simulink library "inp_BCKP"  (R2021b)
settings: Solver=VariableStepAuto  StartTime=0.0  StopTime=10.0  RelTol=1e-3
undefined symbols (not defined in the file): C_TASK_5MS_S, FALSE, KINP_AcoreReadyToSlp_flg_ovrdflg, KINP_AcoreReadyToSlp_flg_ovrdval, KINP_AllowMovThd_OTA_enum_ovrdflg, KINP_AllowMovThd_OTA_enum_ovrdval, KINP_APSAngleTarget_Deg_ovrdflg, KINP_APSAngleTarget_Deg_ovrdval, KINP_APSDecReq_mps2_ovrdflg, KINP_APSDecReq_mps2_ovrdval, KINP_APSDecReqA_flg_ovrdflg, KINP_APSDecReqA_flg_ovrdval, KINP_APSDFLL_cm_ovrdflg, KINP_APSDFLL_cm_ovrdval, KINP_APSDFLR_cm_ovrdflg, KINP_APSDFLR_cm_ovrdval, KINP_APSDRLL_cm_ovrdflg, KINP_APSDRLL_cm_ovrdval, KINP_APSDRLR_cm_ovrdflg, KINP_APSDRLR_cm_ovrdval, KINP_APSExitCondition_enum_ovrdflg, KINP_APSExitCondition_enum_ovrdval, KINP_APSHWVer_enum_ovrdflg, KINP_APSHWVer_enum_ovrdval, KINP_APSProgressPCT_pct_ovrdflg, KINP_APSProgressPCT_pct_ovrdval, KINP_APSPwrReq_enum_ovrdflg, KINP_APSPwrReq_enum_ovrdval, KINP_APSReq_enum_ovrdflg, KINP_APSReq_enum_ovrdval, KINP_APSRQDisplay_enum_ovrdflg, KINP_APSRQDisplay_enum_ovrdval, KINP_APSRqEPASCtrl_flg_ovrdflg, KINP_APSRqEPASCtrl_flg_ovrdval, KINP_APSShiftPosnReq_enum_ovrdval, KINP_APSShiftPosnReq_enum_ovrflg, KINP_APSSpeedCMD_kph_ovrdval, KINP_APSSpeedCMD_kph_ovrflg, KINP_APSStaSystem_enum_ovrdflg, KINP_APSStaSystem_enum_ovrdval, KINP_APSSWVer_enum_ovrdflg, KINP_APSSWVer_enum_ovrdval, KINP_APSVMCReqA_flg_ovrdval, KINP_APSVMCReqA_flg_ovrflg, KINP_APSVRqEPASCtrl_flg_ovrdflg, KINP_APSVRqEPASCtrl_flg_ovrdval, KINP_AuxBattVolmV_mV_ovrdflg, KINP_AuxBattVolmV_mV_ovrdval, KINP_BTConnectSta_enum_ovrdflg, KINP_BTConnectSta_enum_ovrdval, KINP_CAASSta_enum_ovrdflg, KINP_CAASSta_enum_ovrdval, KINP_CAASVMCReqA_flg_ovrdval, KINP_CAASVMCReqA_flg_ovrflg, KINP_CAN1BusOff_flg_ovrdflg, KINP_CAN1BusOff_flg_ovrdval, KINP_CAN2BusOff_flg_ovrdflg, KINP_CAN2BusOff_flg_ovrdval, KINP_CAN3BusOff_flg_ovrdflg, KINP_CAN3BusOff_flg_ovrdval ... (+158)
libraries: FVT_lib x144, hcu_lib x1
(part 8 of 8)

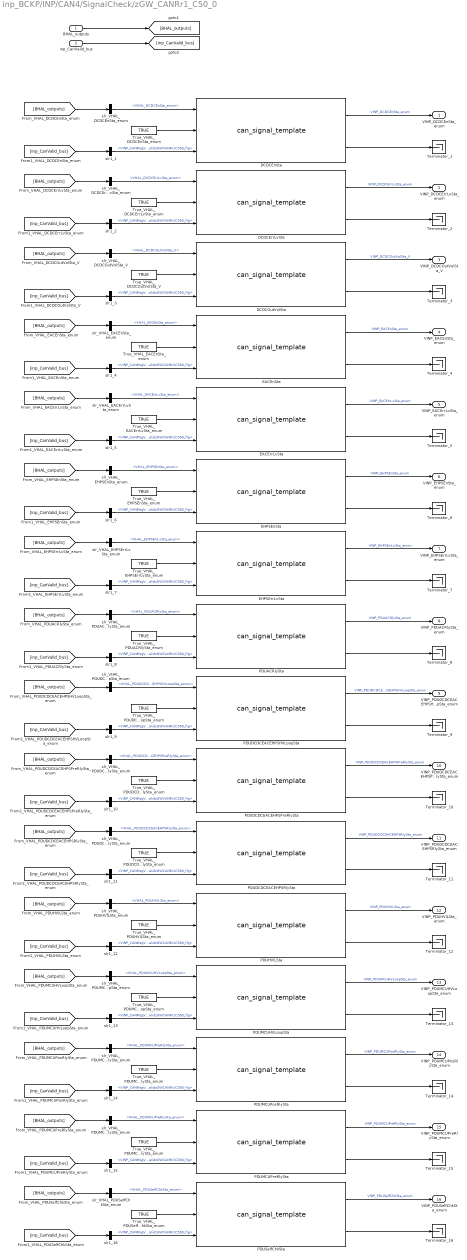
== system inp_BCKP/INP/CAN4/SignalCheck/zGW_CANRr1_C50_0 ==
  BHAL_outputs : Inport
  inp_CanValid_bus : Inport  Port=2
  DCDCEnSta : FVT_lib/inp/can_signal_template  SystemSampleTime=-1  VariantActivationTime=update diagram  Latency=0  AutoFrameSizeCalculation=off
      link override defval: Value=KINP_DCDCEnSta_enum_defval
      link override ovrdflg: Value=KINP_DCDCEnSta_enum_ovrdflg
      link override ovrdval: Value=KINP_DCDCEnSta_enum_ovrdval
  DCDCErrLvSta : FVT_lib/inp/can_signal_template  SystemSampleTime=-1  VariantActivationTime=update diagram  Latency=0  AutoFrameSizeCalculation=off
      link override defval: Value=KINP_DCDCErrLvSta_enum_defval
      link override ovrdflg: Value=KINP_DCDCErrLvSta_enum_ovrdflg
      link override ovrdval: Value=KINP_DCDCErrLvSta_enum_ovrdval
  DCDCOutVolSta : FVT_lib/inp/can_signal_template  SystemSampleTime=-1  VariantActivationTime=update diagram  Latency=0  AutoFrameSizeCalculation=off
      link override defval: Value=KINP_DCDCOutVolSta_V_defval
      link override ovrdflg: Value=KINP_DCDCOutVolSta_V_ovrdflg
      link override ovrdval: Value=KINP_DCDCOutVolSta_V_ovrdval
  EACEnSta : FVT_lib/inp/can_signal_template  SystemSampleTime=-1  VariantActivationTime=update diagram  Latency=0  AutoFrameSizeCalculation=off
      link override defval: Value=KINP_EACEnSta_enum_defval
      link override ovrdflg: Value=KINP_EACEnSta_enum_ovrdflg
      link override ovrdval: Value=KINP_EACEnSta_enum_ovrdval
  EACErrLvSta : FVT_lib/inp/can_signal_template  SystemSampleTime=-1  VariantActivationTime=update diagram  Latency=0  AutoFrameSizeCalculation=off
      link override defval: Value=KINP_EACErrLvSta_enum_defval
      link override ovrdflg: Value=KINP_EACErrLvSta_enum_ovrdflg
      link override ovrdval: Value=KINP_EACErrLvSta_enum_ovrdval
  EHPSEnSta : FVT_lib/inp/can_signal_template  SystemSampleTime=-1  VariantActivationTime=update diagram  Latency=0  AutoFrameSizeCalculation=off
      link override defval: Value=KINP_EHPSEnSta_enum_defval
      link override ovrdflg: Value=KINP_EHPSEnSta_enum_ovrdflg
      link override ovrdval: Value=KINP_EHPSEnSta_enum_ovrdval
  EHPSErrLvSta : FVT_lib/inp/can_signal_template  SystemSampleTime=-1  VariantActivationTime=update diagram  Latency=0  AutoFrameSizeCalculation=off
      link override defval: Value=KINP_EHPSErrLvSta_enum_defval
      link override ovrdflg: Value=KINP_EHPSErrLvSta_enum_ovrdflg
      link override ovrdval: Value=KINP_EHPSErrLvSta_enum_ovrdval
  PDUACRlySta : FVT_lib/inp/can_signal_template  SystemSampleTime=-1  VariantActivationTime=update diagram  Latency=0  AutoFrameSizeCalculation=off
      link override defval: Value=KINP_PDUACRlySta_enum_defval
      link override ovrdflg: Value=KINP_PDUACRlySta_enum_ovrdflg
      link override ovrdval: Value=KINP_PDUACRlySta_enum_ovrdval
  PDUDCDCEACEHPSHVLoopSta : FVT_lib/inp/can_signal_template  SystemSampleTime=-1  VariantActivationTime=update diagram  Latency=0  AutoFrameSizeCalculation=off
      link override defval: Value=KINP_PDUDCDCEACEHPSHVLoopSta_enum_defval
      link override ovrdflg: Value=KINP_PDUDCDCEACEHPSHVLoopSta_enum_ovrdflg
      link override ovrdval: Value=KINP_PDUDCDCEACEHPSHVLoopSta_enum_ovrdval
  PDUDCDCEACEHPSPreRlySta : FVT_lib/inp/can_signal_template  SystemSampleTime=-1  VariantActivationTime=update diagram  Latency=0  AutoFrameSizeCalculation=off
      link override defval: Value=KINP_PDUDCDCEACEHPSPreRlySta_enum_defval
      link override ovrdflg: Value=KINP_PDUDCDCEACEHPSPreRlySta_enum_ovrdflg
      link override ovrdval: Value=KINP_PDUDCDCEACEHPSPreRlySta_enum_ovrdval
  PDUDCDCEACEHPSRlySta : FVT_lib/inp/can_signal_template  SystemSampleTime=-1  VariantActivationTime=update diagram  Latency=0  AutoFrameSizeCalculation=off
      link override defval: Value=KINP_PDUDCDCEACEHPSRlySta_enum_defval
      link override ovrdflg: Value=KINP_PDUDCDCEACEHPSRlySta_enum_ovrdflg
      link override ovrdval: Value=KINP_PDUDCDCEACEHPSRlySta_enum_ovrdval
  PDUHVILSta : FVT_lib/inp/can_signal_template  SystemSampleTime=-1  VariantActivationTime=update diagram  Latency=0  AutoFrameSizeCalculation=off
      link override defval: Value=KINP_PDUHVILSta_enum_defval
      link override ovrdflg: Value=KINP_PDUHVILSta_enum_ovrdflg
      link override ovrdval: Value=KINP_PDUHVILSta_enum_ovrdval
  PDUMCUHVLoopSta : FVT_lib/inp/can_signal_template  SystemSampleTime=-1  VariantActivationTime=update diagram  Latency=0  AutoFrameSizeCalculation=off
      link override defval: Value=KINP_PDUMCUHVLoopSta_enum_defval
      link override ovrdflg: Value=KINP_PDUMCUHVLoopSta_enum_ovrdflg
      link override ovrdval: Value=KINP_PDUMCUHVLoopSta_enum_ovrdval
  PDUMCUPosRlySta : FVT_lib/inp/can_signal_template  SystemSampleTime=-1  VariantActivationTime=update diagram  Latency=0  AutoFrameSizeCalculation=off
      link override defval: Value=KINP_PDUMCUPosRlySta_enum_defval
      link override ovrdflg: Value=KINP_PDUMCUPosRlySta_enum_ovrdflg
      link override ovrdval: Value=KINP_PDUMCUPosRlySta_enum_ovrdval
  PDUMCUPreRlySta : FVT_lib/inp/can_signal_template  SystemSampleTime=-1  VariantActivationTime=update diagram  Latency=0  AutoFrameSizeCalculation=off
      link override defval: Value=KINP_PDUMCUPreRlySta_enum_defval
      link override ovrdflg: Value=KINP_PDUMCUPreRlySta_enum_ovrdflg
      link override ovrdval: Value=KINP_PDUMCUPreRlySta_enum_ovrdval
  PDUSelfChkSta : FVT_lib/inp/can_signal_template  SystemSampleTime=-1  VariantActivationTime=update diagram  Latency=0  AutoFrameSizeCalculation=off
      link override defval: Value=KINP_PDUSelfChkSta_enum_defval
      link override ovrdflg: Value=KINP_PDUSelfChkSta_enum_ovrdflg
      link override ovrdval: Value=KINP_PDUSelfChkSta_enum_ovrdval
  Terminator_{1..16} (16 alike) : Terminator
  True_VHAL_DCDCEnSta_enum : Constant  Value=TRUE  OutDataTypeStr=boolean
  True_VHAL_DCDCErrLvSta_enum : Constant  Value=TRUE  OutDataTypeStr=boolean
  True_VHAL_DCDCOutVolSta_V : Constant  Value=TRUE  OutDataTypeStr=boolean
  True_VHAL_EACEnSta_enum : Constant  Value=TRUE  OutDataTypeStr=boolean
  True_VHAL_EACErrLvSta_enum : Constant  Value=TRUE  OutDataTypeStr=boolean
  True_VHAL_EHPSEnSta_enum : Constant  Value=TRUE  OutDataTypeStr=boolean
  True_VHAL_EHPSErrLvSta_enum : Constant  Value=TRUE  OutDataTypeStr=boolean
  True_VHAL_PDUACRlySta_enum : Constant  Value=TRUE  OutDataTypeStr=boolean
  True_VHAL_PDUDCDCEACEHPSHVLoopSta_enum : Constant  Value=TRUE  OutDataTypeStr=boolean
  True_VHAL_PDUDCDCEACEHPSPreRlySta_enum : Constant  Value=TRUE  OutDataTypeStr=boolean
  True_VHAL_PDUDCDCEACEHPSRlySta_enum : Constant  Value=TRUE  OutDataTypeStr=boolean
  True_VHAL_PDUHVILSta_enum : Constant  Value=TRUE  OutDataTypeStr=boolean
  True_VHAL_PDUMCUHVLoopSta_enum : Constant  Value=TRUE  OutDataTypeStr=boolean
  True_VHAL_PDUMCUPosRlySta_enum : Constant  Value=TRUE  OutDataTypeStr=boolean
  True_VHAL_PDUMCUPreRlySta_enum : Constant  Value=TRUE  OutDataTypeStr=boolean
  True_VHAL_PDUSelfChkSta_enum : Constant  Value=TRUE  OutDataTypeStr=boolean
  slr1_{1..16} (16 alike) : BusSelector  OutputSignals=VINP_CANMsgValidzGWCANRr1C500_flg
  slr_VHAL_DCDCEnSta_enum : BusSelector  OutputSignals=VHAL_DCDCEnSta_enum
  slr_VHAL_DCDCErrLvSta_enum : BusSelector  OutputSignals=VHAL_DCDCErrLvSta_enum
  slr_VHAL_DCDCOutVolSta_V : BusSelector  OutputSignals=VHAL_DCDCOutVolSta_V
  slr_VHAL_EACEnSta_enum : BusSelector  OutputSignals=VHAL_EACEnSta_enum
  slr_VHAL_EACErrLvSta_enum : BusSelector  OutputSignals=VHAL_EACErrLvSta_enum
  slr_VHAL_EHPSEnSta_enum : BusSelector  OutputSignals=VHAL_EHPSEnSta_enum
  slr_VHAL_EHPSErrLvSta_enum : BusSelector  OutputSignals=VHAL_EHPSErrLvSta_enum
  slr_VHAL_PDUACRlySta_enum : BusSelector  OutputSignals=VHAL_PDUACRlySta_enum
  slr_VHAL_PDUDCDCEACEHPSHVLoopSta_enum : BusSelector  OutputSignals=VHAL_PDUDCDCEACEHPSHVLoopSta_enum
  slr_VHAL_PDUDCDCEACEHPSPreRlySta_enum : BusSelector  OutputSignals=VHAL_PDUDCDCEACEHPSPreRlySta_enum
  slr_VHAL_PDUDCDCEACEHPSRlySta_enum : BusSelector  OutputSignals=VHAL_PDUDCDCEACEHPSRlySta_enum
  slr_VHAL_PDUHVILSta_enum : BusSelector  OutputSignals=VHAL_PDUHVILSta_enum
  slr_VHAL_PDUMCUHVLoopSta_enum : BusSelector  OutputSignals=VHAL_PDUMCUHVLoopSta_enum
  slr_VHAL_PDUMCUPosRlySta_enum : BusSelector  OutputSignals=VHAL_PDUMCUPosRlySta_enum
  slr_VHAL_PDUMCUPreRlySta_enum : BusSelector  OutputSignals=VHAL_PDUMCUPreRlySta_enum
  slr_VHAL_PDUSelfChkSta_enum : BusSelector  OutputSignals=VHAL_PDUSelfChkSta_enum
  VINP_DCDCEnSta_enum : Outport
  VINP_DCDCErrLvSta_enum : Outport  Port=2
  VINP_DCDCOutVolSta_V : Outport  Port=3
  VINP_EACEnSta_enum : Outport  Port=4
  VINP_EACErrLvSta_enum : Outport  Port=5
  VINP_EHPSEnSta_enum : Outport  Port=6
  VINP_EHPSErrLvSta_enum : Outport  Port=7
  VINP_PDUACRlySta_enum : Outport  Port=8
  VINP_PDUDCDCEACEHPSHVLoopSta_enum : Outport  Port=9
  VINP_PDUDCDCEACEHPSPreRlySta_enum : Outport  Port=10
  VINP_PDUDCDCEACEHPSRlySta_enum : Outport  Port=11
  VINP_PDUHVILSta_enum : Outport  Port=12
  VINP_PDUMCUHVLoopSta_enum : Outport  Port=13
  VINP_PDUMCUPosRlySta_enum : Outport  Port=14
  VINP_PDUMCUPreRlySta_enum : Outport  Port=15
  VINP_PDUSelfChkSta_enum : Outport  Port=16
  wires:
  BHAL_outputs/1 -> [BHAL_outputs]
  inp_CanValid_bus/1 -> [inp_CanValid_bus]
  [BHAL_outputs] -> slr_VHAL_DCDCEnSta_enum/1
  slr_VHAL_DCDCEnSta_enum/1 -> DCDCEnSta/1  "<VHAL_DCDCEnSta_enum>"
  True_VHAL_DCDCEnSta_enum/1 -> DCDCEnSta/2
  [inp_CanValid_bus] -> slr1_1/1
  slr1_1/1 -> DCDCEnSta/3  "<VINP_CANMsgValidzGWCANRr1C500_flg>"
  DCDCEnSta/1 -> VINP_DCDCEnSta_enum/1  "VINP_DCDCEnSta_enum"
  DCDCEnSta/2 -> Terminator_1/1
  [BHAL_outputs] -> slr_VHAL_DCDCErrLvSta_enum/1
  slr_VHAL_DCDCErrLvSta_enum/1 -> DCDCErrLvSta/1  "<VHAL_DCDCErrLvSta_enum>"
  True_VHAL_DCDCErrLvSta_enum/1 -> DCDCErrLvSta/2
  [inp_CanValid_bus] -> slr1_2/1
  slr1_2/1 -> DCDCErrLvSta/3  "<VINP_CANMsgValidzGWCANRr1C500_flg>"
  DCDCErrLvSta/1 -> VINP_DCDCErrLvSta_enum/1  "VINP_DCDCErrLvSta_enum"
  DCDCErrLvSta/2 -> Terminator_2/1
  [BHAL_outputs] -> slr_VHAL_DCDCOutVolSta_V/1
  slr_VHAL_DCDCOutVolSta_V/1 -> DCDCOutVolSta/1  "<VHAL_DCDCOutVolSta_V>"
  True_VHAL_DCDCOutVolSta_V/1 -> DCDCOutVolSta/2
  [inp_CanValid_bus] -> slr1_3/1
  slr1_3/1 -> DCDCOutVolSta/3  "<VINP_CANMsgValidzGWCANRr1C500_flg>"
  DCDCOutVolSta/1 -> VINP_DCDCOutVolSta_V/1  "VINP_DCDCOutVolSta_V"
  DCDCOutVolSta/2 -> Terminator_3/1
  [BHAL_outputs] -> slr_VHAL_EACEnSta_enum/1
  slr_VHAL_EACEnSta_enum/1 -> EACEnSta/1  "<VHAL_EACEnSta_enum>"
  True_VHAL_EACEnSta_enum/1 -> EACEnSta/2
  [inp_CanValid_bus] -> slr1_4/1
  slr1_4/1 -> EACEnSta/3  "<VINP_CANMsgValidzGWCANRr1C500_flg>"
  EACEnSta/1 -> VINP_EACEnSta_enum/1  "VINP_EACEnSta_enum"
  EACEnSta/2 -> Terminator_4/1
  [BHAL_outputs] -> slr_VHAL_EACErrLvSta_enum/1
  slr_VHAL_EACErrLvSta_enum/1 -> EACErrLvSta/1  "<VHAL_EACErrLvSta_enum>"
  True_VHAL_EACErrLvSta_enum/1 -> EACErrLvSta/2
  [inp_CanValid_bus] -> slr1_5/1
  slr1_5/1 -> EACErrLvSta/3  "<VINP_CANMsgValidzGWCANRr1C500_flg>"
  EACErrLvSta/1 -> VINP_EACErrLvSta_enum/1  "VINP_EACErrLvSta_enum"
  EACErrLvSta/2 -> Terminator_5/1
  [BHAL_outputs] -> slr_VHAL_EHPSEnSta_enum/1
  slr_VHAL_EHPSEnSta_enum/1 -> EHPSEnSta/1  "<VHAL_EHPSEnSta_enum>"
  True_VHAL_EHPSEnSta_enum/1 -> EHPSEnSta/2
  [inp_CanValid_bus] -> slr1_6/1
  slr1_6/1 -> EHPSEnSta/3  "<VINP_CANMsgValidzGWCANRr1C500_flg>"
  EHPSEnSta/1 -> VINP_EHPSEnSta_enum/1  "VINP_EHPSEnSta_enum"
  EHPSEnSta/2 -> Terminator_6/1
  [BHAL_outputs] -> slr_VHAL_EHPSErrLvSta_enum/1
  slr_VHAL_EHPSErrLvSta_enum/1 -> EHPSErrLvSta/1  "<VHAL_EHPSErrLvSta_enum>"
  True_VHAL_EHPSErrLvSta_enum/1 -> EHPSErrLvSta/2
  [inp_CanValid_bus] -> slr1_7/1
  slr1_7/1 -> EHPSErrLvSta/3  "<VINP_CANMsgValidzGWCANRr1C500_flg>"
  EHPSErrLvSta/1 -> VINP_EHPSErrLvSta_enum/1  "VINP_EHPSErrLvSta_enum"
  EHPSErrLvSta/2 -> Terminator_7/1
  [BHAL_outputs] -> slr_VHAL_PDUACRlySta_enum/1
  slr_VHAL_PDUACRlySta_enum/1 -> PDUACRlySta/1  "<VHAL_PDUACRlySta_enum>"
  True_VHAL_PDUACRlySta_enum/1 -> PDUACRlySta/2
  [inp_CanValid_bus] -> slr1_8/1
  slr1_8/1 -> PDUACRlySta/3  "<VINP_CANMsgValidzGWCANRr1C500_flg>"
  PDUACRlySta/1 -> VINP_PDUACRlySta_enum/1  "VINP_PDUACRlySta_enum"
  PDUACRlySta/2 -> Terminator_8/1
  [BHAL_outputs] -> slr_VHAL_PDUDCDCEACEHPSHVLoopSta_enum/1
  slr_VHAL_PDUDCDCEACEHPSHVLoopSta_enum/1 -> PDUDCDCEACEHPSHVLoopSta/1  "<VHAL_PDUDCDCEACEHPSHVLoopSta_enum>"
  True_VHAL_PDUDCDCEACEHPSHVLoopSta_enum/1 -> PDUDCDCEACEHPSHVLoopSta/2
  [inp_CanValid_bus] -> slr1_9/1
  slr1_9/1 -> PDUDCDCEACEHPSHVLoopSta/3  "<VINP_CANMsgValidzGWCANRr1C500_flg>"
  PDUDCDCEACEHPSHVLoopSta/1 -> VINP_PDUDCDCEACEHPSHVLoopSta_enum/1  "VINP_PDUDCDCEACEHPSHVLoopSta_enum"
  PDUDCDCEACEHPSHVLoopSta/2 -> Terminator_9/1
  [BHAL_outputs] -> slr_VHAL_PDUDCDCEACEHPSPreRlySta_enum/1
  slr_VHAL_PDUDCDCEACEHPSPreRlySta_enum/1 -> PDUDCDCEACEHPSPreRlySta/1  "<VHAL_PDUDCDCEACEHPSPreRlySta_enum>"
  True_VHAL_PDUDCDCEACEHPSPreRlySta_enum/1 -> PDUDCDCEACEHPSPreRlySta/2
  [inp_CanValid_bus] -> slr1_10/1
  slr1_10/1 -> PDUDCDCEACEHPSPreRlySta/3  "<VINP_CANMsgValidzGWCANRr1C500_flg>"
  PDUDCDCEACEHPSPreRlySta/1 -> VINP_PDUDCDCEACEHPSPreRlySta_enum/1  "VINP_PDUDCDCEACEHPSPreRlySta_enum"
  PDUDCDCEACEHPSPreRlySta/2 -> Terminator_10/1
  [BHAL_outputs] -> slr_VHAL_PDUDCDCEACEHPSRlySta_enum/1
  slr_VHAL_PDUDCDCEACEHPSRlySta_enum/1 -> PDUDCDCEACEHPSRlySta/1  "<VHAL_PDUDCDCEACEHPSRlySta_enum>"
  True_VHAL_PDUDCDCEACEHPSRlySta_enum/1 -> PDUDCDCEACEHPSRlySta/2
  [inp_CanValid_bus] -> slr1_11/1
  slr1_11/1 -> PDUDCDCEACEHPSRlySta/3  "<VINP_CANMsgValidzGWCANRr1C500_flg>"
  PDUDCDCEACEHPSRlySta/1 -> VINP_PDUDCDCEACEHPSRlySta_enum/1  "VINP_PDUDCDCEACEHPSRlySta_enum"
  PDUDCDCEACEHPSRlySta/2 -> Terminator_11/1
  [BHAL_outputs] -> slr_VHAL_PDUHVILSta_enum/1
  slr_VHAL_PDUHVILSta_enum/1 -> PDUHVILSta/1  "<VHAL_PDUHVILSta_enum>"
  True_VHAL_PDUHVILSta_enum/1 -> PDUHVILSta/2
  [inp_CanValid_bus] -> slr1_12/1
  slr1_12/1 -> PDUHVILSta/3  "<VINP_CANMsgValidzGWCANRr1C500_flg>"
  PDUHVILSta/1 -> VINP_PDUHVILSta_enum/1  "VINP_PDUHVILSta_enum"
  PDUHVILSta/2 -> Terminator_12/1
  [BHAL_outputs] -> slr_VHAL_PDUMCUHVLoopSta_enum/1
  slr_VHAL_PDUMCUHVLoopSta_enum/1 -> PDUMCUHVLoopSta/1  "<VHAL_PDUMCUHVLoopSta_enum>"
  True_VHAL_PDUMCUHVLoopSta_enum/1 -> PDUMCUHVLoopSta/2
  [inp_CanValid_bus] -> slr1_13/1
  slr1_13/1 -> PDUMCUHVLoopSta/3  "<VINP_CANMsgValidzGWCANRr1C500_flg>"
  PDUMCUHVLoopSta/1 -> VINP_PDUMCUHVLoopSta_enum/1  "VINP_PDUMCUHVLoopSta_enum"
  PDUMCUHVLoopSta/2 -> Terminator_13/1
  [BHAL_outputs] -> slr_VHAL_PDUMCUPosRlySta_enum/1
  slr_VHAL_PDUMCUPosRlySta_enum/1 -> PDUMCUPosRlySta/1  "<VHAL_PDUMCUPosRlySta_enum>"
  True_VHAL_PDUMCUPosRlySta_enum/1 -> PDUMCUPosRlySta/2
  [inp_CanValid_bus] -> slr1_14/1
  slr1_14/1 -> PDUMCUPosRlySta/3  "<VINP_CANMsgValidzGWCANRr1C500_flg>"
  PDUMCUPosRlySta/1 -> VINP_PDUMCUPosRlySta_enum/1  "VINP_PDUMCUPosRlySta_enum"
  PDUMCUPosRlySta/2 -> Terminator_14/1
  [BHAL_outputs] -> slr_VHAL_PDUMCUPreRlySta_enum/1
  slr_VHAL_PDUMCUPreRlySta_enum/1 -> PDUMCUPreRlySta/1  "<VHAL_PDUMCUPreRlySta_enum>"
  True_VHAL_PDUMCUPreRlySta_enum/1 -> PDUMCUPreRlySta/2
  [inp_CanValid_bus] -> slr1_15/1
  slr1_15/1 -> PDUMCUPreRlySta/3  "<VINP_CANMsgValidzGWCANRr1C500_flg>"
  PDUMCUPreRlySta/1 -> VINP_PDUMCUPreRlySta_enum/1  "VINP_PDUMCUPreRlySta_enum"
  PDUMCUPreRlySta/2 -> Terminator_15/1
  [BHAL_outputs] -> slr_VHAL_PDUSelfChkSta_enum/1
  slr_VHAL_PDUSelfChkSta_enum/1 -> PDUSelfChkSta/1  "<VHAL_PDUSelfChkSta_enum>"
  True_VHAL_PDUSelfChkSta_enum/1 -> PDUSelfChkSta/2
  [inp_CanValid_bus] -> slr1_16/1
  slr1_16/1 -> PDUSelfChkSta/3  "<VINP_CANMsgValidzGWCANRr1C500_flg>"
  PDUSelfChkSta/1 -> VINP_PDUSelfChkSta_enum/1  "VINP_PDUSelfChkSta_enum"
  PDUSelfChkSta/2 -> Terminator_16/1
